simulink model "flightController"  (R2020b)
settings: Solver=ode3  StartTime=0.0  StopTime=10.0  FixedStep=Ts  RelTol=1e-3
undefined symbols (not defined in the file): DiscIntNeverNeededParam, Discrete, Estimator, g, init, Time, Ts
libraries: sharedtransform x3, pid_lib x2, aerolibconvert2 x1, ctrlSharedLib x1
settings Model: Creator=dbell44  LastModifiedBy=dbell44
settings OptimizationCC: DefaultParameterBehavior=Inlined  GainParamInheritBuiltInType=on  UseFloatMulNetSlope=on  DefaultUnderspecifiedDataType=single  UseSpecifiedMinMax=on  InlineInvariantSignals=on  PassReuseOutputArgsAs=Individual arguments  NoFixptDivByZeroProtection=on  EfficientFloat2IntCast=on  LifeSpan=1  OptimizeBlockOrder=speed  DifferentSizesBufferReuse=on  EfficientTunableParamExpr=on
settings DebuggingCC: ParameterTunabilityLossMsg=error  SFUnexpectedBacktrackingDiag=warning  SFNoUnconditionalDefaultTransitionDiag=warning
settings HardwareCC: ProdBitPerPointer=32  ProdBitPerSizeT=32  ProdBitPerPtrDiffT=32  ProdLargestAtomicInteger=Long  ProdLargestAtomicFloat=Double  ProdWordSize=32  ProdLongLongMode=on  ProdHWDeviceType=ARM Compatible->ARM Cortex-M
settings SFSimCC: MATLABDynamicMemAlloc=off
settings RTWCC: Description=Embedded Coder  SystemTargetFile=ert.tlc  GenCodeOnly=on  TemplateMakefile=ert_default_tmf  GenerateReport=on  BuildConfiguration=Faster Runs  LaunchReport=on  GenerateCodeMetricsReport=on
settings CodeAppCC: ForceParamTrailComments=on  IgnoreCustomStorageClasses=off  OperatorAnnotations=on  SimulinkDataObjDesc=on  SFDataObjDesc=on  CustomSymbolStrGlobalVar=rt$N$M  CustomSymbolStrType=$N$M  CustomSymbolStrFcn=$N$M$F  CustomSymbolStrMacro=$N$M  InsertBlockDesc=on  EnableCustomComments=on
settings ERTTargetCC: TargetLangStandard=C99 (ISO)  GenerateSampleERTMain=on  IncludeMdlTerminateFcn=off  CombineSignalStateStructs=on  SuppressErrorStatus=on  SupportAbsoluteTime=off  CodeInterfacePackaging=Reusable function  SupportNonFinite=off  SupportComplex=off  InlinedParameterPlacement=NonHierarchical  ERTCustomFileTemplate=example_file_process.tlc  ERTFilePackagingFormat=CompactWithDataFile

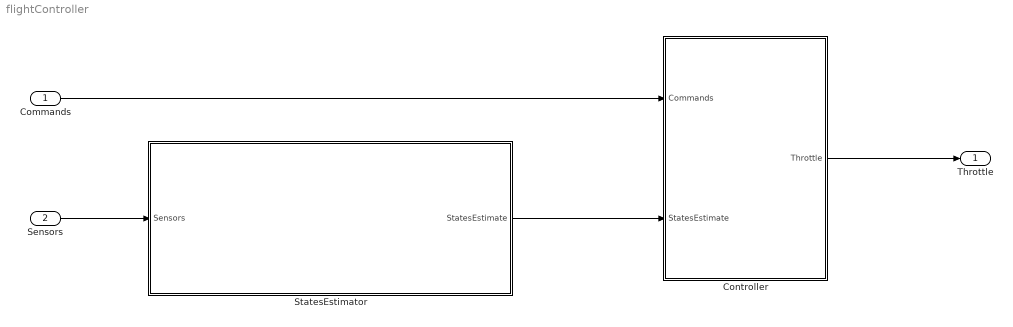
== system flightController ==
  Commands : Inport  OutDataTypeStr=Bus: command_t
  Sensors : Inport  Port=2  OutDataTypeStr=Bus: sensor_data_t
  Controller : Subsystem  TreatAsAtomicUnit=on
  StatesEstimator : Subsystem  TreatAsAtomicUnit=on
  Throttle : Outport
  wires:
  Sensors/1 -> StatesEstimator/1(Sensors)
  StatesEstimator/1(StatesEstimate) -> Controller/2(StatesEstimate)
  Commands/1 -> Controller/1(Commands)
  Controller/1(Throttle) -> Throttle/1

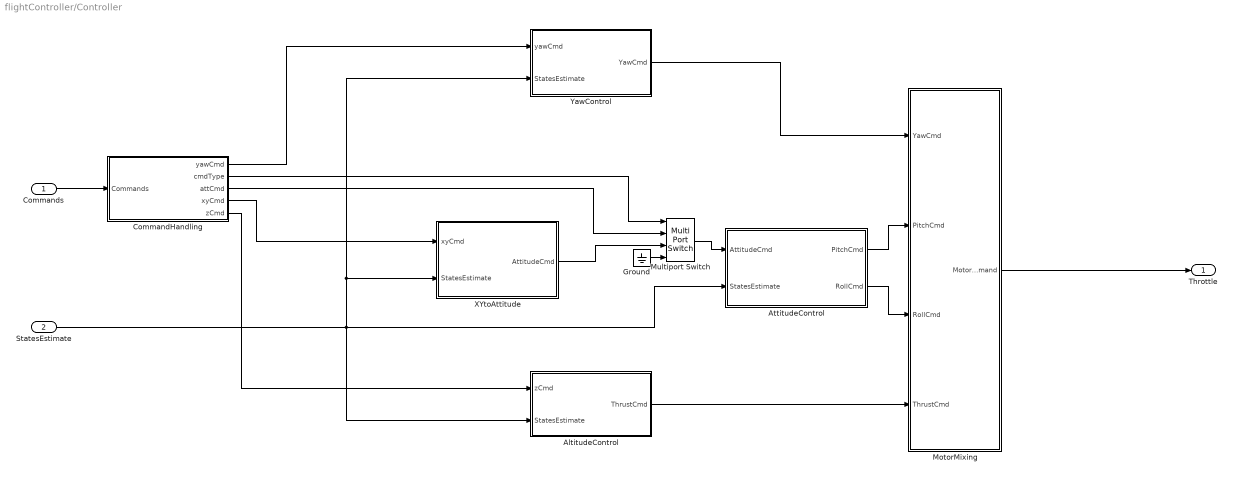
== system flightController/Controller ==
  Commands : Inport
  StatesEstimate : Inport  Port=2  OutDataTypeStr=Bus: states_estimate_t
  AltitudeControl : Subsystem
  AttitudeControl : Subsystem
  CommandHandling : Subsystem
  Ground : Ground
  MotorMixing : Subsystem
  Multiport Switch : MultiPortSwitch
  XYtoAttitude : Subsystem
  YawControl : Subsystem
  Throttle : Outport
  wires:
  StatesEstimate/1 -> YawControl/2(StatesEstimate), XYtoAttitude/2(StatesEstimate), AltitudeControl/2(StatesEstimate), AttitudeControl/2(StatesEstimate)
  AltitudeControl/1(ThrustCmd) -> MotorMixing/4(ThrustCmd)
  MotorMixing/1(MotorCommand) -> Throttle/1
  YawControl/1(YawCmd) -> MotorMixing/1(YawCmd)
  AttitudeControl/1(PitchCmd) -> MotorMixing/2(PitchCmd)
  AttitudeControl/2(RollCmd) -> MotorMixing/3(RollCmd)
  XYtoAttitude/1(AttitudeCmd) -> Multiport Switch/3
  Commands/1 -> CommandHandling/1(Commands)
  CommandHandling/1(yawCmd) -> YawControl/1(yawCmd)
  CommandHandling/5(zCmd) -> AltitudeControl/1(zCmd)
  CommandHandling/4(xyCmd) -> XYtoAttitude/1(xyCmd)
  CommandHandling/3(attCmd) -> Multiport Switch/2
  CommandHandling/2(cmdType) -> Multiport Switch/1
  Multiport Switch/1 -> AttitudeControl/1(AttitudeCmd)
  Ground/1 -> Multiport Switch/4

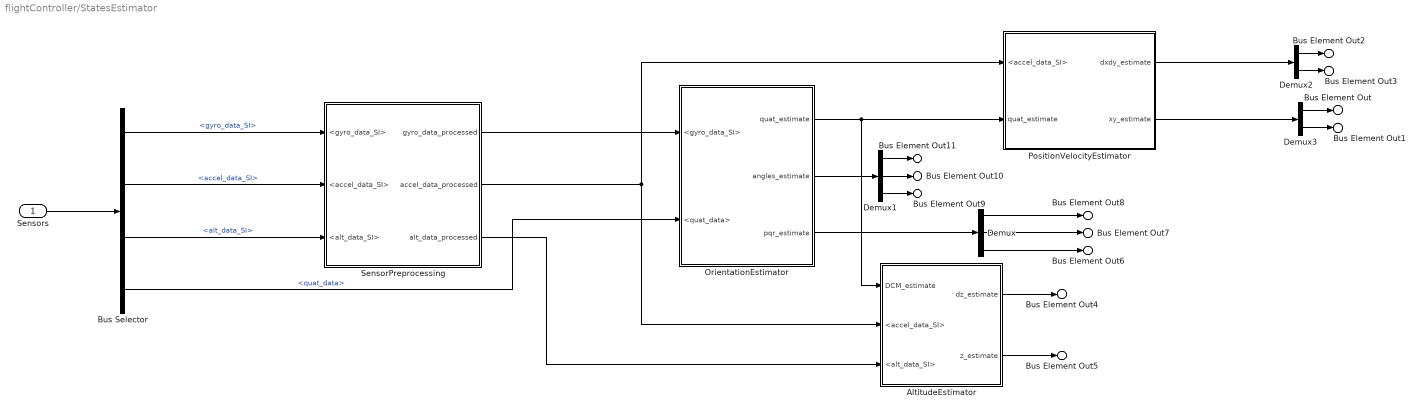
== system flightController/StatesEstimator ==
  Sensors : Inport  OutDataTypeStr=Bus: sensor_data_t
  AltitudeEstimator : Subsystem
  Bus Selector : BusSelector  OutputSignals=gyro_data_SI,accel_data_SI,alt_data_SI,quat_data
  Demux : Demux  Outputs=3
  Demux1 : Demux  Outputs=3
  Demux2 : Demux  Outputs=2
  Demux3 : Demux  Outputs=2
  OrientationEstimator : Subsystem
  PositionVelocityEstimator : Subsystem
  SensorPreprocessing : Subsystem
  Bus Element Out : Outport  PortName=StatesEstimate  Element=x
  Bus Element Out1 : Outport  PortName=StatesEstimate  Element=y
  Bus Element Out2 : Outport  PortName=StatesEstimate  Element=dx
  Bus Element Out3 : Outport  PortName=StatesEstimate  Element=dy
  Bus Element Out4 : Outport  PortName=StatesEstimate  Element=dz
  Bus Element Out5 : Outport  PortName=StatesEstimate  Element=z
  Bus Element Out6 : Outport  PortName=StatesEstimate  Element=r
  Bus Element Out7 : Outport  PortName=StatesEstimate  Element=q
  Bus Element Out8 : Outport  PortName=StatesEstimate  Element=p
  Bus Element Out9 : Outport  PortName=StatesEstimate  Element=roll
  Bus Element Out10 : Outport  PortName=StatesEstimate  Element=pitch
  Bus Element Out11 : Outport  PortName=StatesEstimate  Element=yaw
  wires:
  Sensors/1 -> Bus Selector/1
  Bus Selector/3 -> SensorPreprocessing/3(<alt_data_SI>)  "<alt_data_SI>"
  PositionVelocityEstimator/1(dxdy_estimate) -> Demux2/1
  PositionVelocityEstimator/2(xy_estimate) -> Demux3/1
  OrientationEstimator/1(quat_estimate) -> AltitudeEstimator/1(DCM_estimate), PositionVelocityEstimator/2(quat_estimate)
  Bus Selector/1 -> SensorPreprocessing/1(<gyro_data_SI>)  "<gyro_data_SI>"
  OrientationEstimator/2(angles_estimate) -> Demux1/1
  Demux1/2 -> Bus Element Out10/1
  AltitudeEstimator/2(z_estimate) -> Bus Element Out5/1
  Demux3/1 -> Bus Element Out/1
  Demux3/2 -> Bus Element Out1/1
  Demux2/1 -> Bus Element Out2/1
  Demux2/2 -> Bus Element Out3/1
  Demux1/3 -> Bus Element Out9/1
  Demux1/1 -> Bus Element Out11/1
  OrientationEstimator/3(pqr_estimate) -> Demux/1
  Demux/1 -> Bus Element Out8/1
  Demux/2 -> Bus Element Out7/1
  Demux/3 -> Bus Element Out6/1
  SensorPreprocessing/2(accel_data_processed) -> AltitudeEstimator/2(<accel_data_SI>), PositionVelocityEstimator/1(<accel_data_SI>)
  Bus Selector/2 -> SensorPreprocessing/2(<accel_data_SI>)  "<accel_data_SI>"
  SensorPreprocessing/1(gyro_data_processed) -> OrientationEstimator/1(<gyro_data_SI>)
  SensorPreprocessing/3(alt_data_processed) -> AltitudeEstimator/3(<alt_data_SI>)
  Bus Selector/4 -> OrientationEstimator/2(<quat_data>)  "<quat_data>"
  AltitudeEstimator/1(dz_estimate) -> Bus Element Out4/1

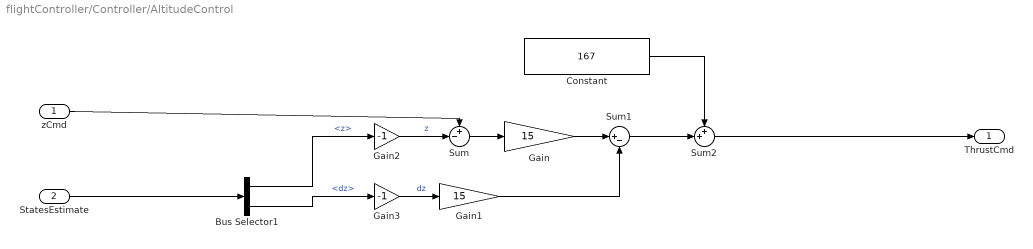
== system flightController/Controller/AltitudeControl ==
  zCmd : Inport
  StatesEstimate : Inport  Port=2
  Bus Selector1 : BusSelector  OutputSignals=z,dz
  Constant : Constant  Value=167
  Gain : Gain  Gain=15
  Gain1 : Gain  Gain=15
  Gain2 : Gain  Gain=-1
  Gain3 : Gain  Gain=-1
  Sum : Sum  Inputs=+-|
  Sum1 : Sum  Inputs=|+-
  Sum2 : Sum  Inputs=++|
  ThrustCmd : Outport
  wires:
  Gain3/1 -> Gain1/1  "dz"
  Bus Selector1/1 -> Gain2/1  "<z>"
  Gain2/1 -> Sum/2  "z"
  Gain1/1 -> Sum1/2
  Constant/1 -> Sum2/1
  Sum2/1 -> ThrustCmd/1
  Sum/1 -> Gain/1
  Bus Selector1/2 -> Gain3/1  "<dz>"
  Gain/1 -> Sum1/1
  StatesEstimate/1 -> Bus Selector1/1
  zCmd/1 -> Sum/1
  Sum1/1 -> Sum2/2

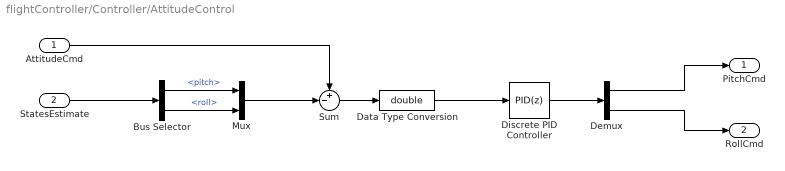
== system flightController/Controller/AttitudeControl ==
  AttitudeCmd : Inport
  StatesEstimate : Inport  Port=2
  Bus Selector : BusSelector  OutputSignals=pitch,roll
  Data Type Conversion : DataTypeConversion  OutDataTypeStr=double
  Demux : Demux  Outputs=2
  Discrete PID Controller : pid_lib/PID Controller  Controller=PID  Form=Parallel  TimeDomain=Discrete-time  UseExternalTs=off  SampleTime=-1  IntegratorMethod=Forward Euler  FilterMethod=Forward Euler  ControllerParametersSource=internal  P=5  I=5  D=3  UseFilter=off  N=100  TunerSelectOption=Transfer Function Based (PID Tuner App)  InitialConditionSource=internal  InitialConditionForIntegrator=0  InitialConditionForFilter=0  DifferentiatorICPrevScaledInput=0  ExternalReset=none  TrackingMode=off  Kt=1  LimitOutput=off  SatLimitsSource=internal  UpperSaturationLimit=inf  LowerSaturationLimit=-inf  LinearizeAsGain=off  AntiWindupMode=none  Kb=1  POutMin=[]  POutMax=[]  IOutMin=[]  IOutMax=[]  DOutMin=[]  DOutMax=[]  NOutMin=[]  NOutMax=[]  SumOutMin=[]  SumOutMax=[]  SaturationOutMin=[]  SaturationOutMax=[]  PParamMin=[]  PParamMax=[]  IParamMin=[]  IParamMax=[]  DParamMin=[]  DParamMax=[]  NParamMin=[]  NParamMax=[]  KbParamMin=[]  KbParamMax=[]  KtParamMin=[]  KtParamMax=[]  KbOutMin=[]  KbOutMax=[]  KtOutMin=[]  KtOutMax=[]  IntegratorOutMin=[]  IntegratorOutMax=[]  FilterOutMin=[]  FilterOutMax=[]  SumI1OutMin=[]  SumI1OutMax=[]  SumI2OutMin=[]  SumI2OutMax=[]  SumI3OutMin=[]  SumI3OutMax=[]  SumI4OutMin=[]  SumI4OutMax=[]  SumDOutMin=[]  SumDOutMax=[]  DifferentiatorOutMin=[]  DifferentiatorOutMax=[]  FilterDiffOutCoefMin=[]  FilterDiffOutCoefMax=[]  ReciprocalOutMin=[]  ReciprocalOutMax=[]  SumDenOutMin=[]  SumDenOutMax=[]  SumNumOutMin=[]  SumNumOutMax=[]  DivideOutMin=[]  DivideOutMax=[]  UdiffTsProdOutMin=[]  UdiffTsProdOutMax=[]  NTsProdOutMin=[]  NTsProdOutMax=[]  UintegralTsProdOutMin=[]  UintegralTsProdOutMax=[]  UngainTsProdOutMin=[]  UngainTsProdOutMax=[]  IntegratorContinuousStateAttributes=''  IntegratorStateMustResolveToSignalObject=off  IntegratorRTWStateStorageClass=Auto  FilterContinuousStateAttributes=''  FilterStateMustResolveToSignalObject=off  FilterRTWStateStorageClass=Auto  ParallelPVariant=InternalParameters  IdealPVariant=Disabled  IVariant=InternalParameters  DVariant=InternalParameters  IntegratorVariant=Discrete  SatVariant=Disabled  AWVariant=Passthrough  PCopyVariant=Disabled  TRVariant=Disabled  FdbkBlocksVariant=Forward  IdealPFdbkVariant=Disabled  SatFdbkVariant=Disabled  DerivativeFilterVariant=Differentiator  NVariant=Passthrough  NCopyVariant=Disabled_SignalSpec  FilterICVariant=InternalICsDifferentiator  IntegratorICVariant=InternalICs  ExternalResetVariant=Disabled  TRSumVariant=Passthrough  SumFdbkVariant=Disabled  SumVariant=Sum_PID  TsampFilterVariant=InternalTs  TsampNgainVariant=Passthrough  TsampIntegralVariant=Passthrough  ExternalSaturationOutDataTypeStr=Inherit: Same as second input
  Mux : Mux  Inputs=2
  Sum : Sum  Inputs=+-|
  PitchCmd : Outport
  RollCmd : Outport  Port=2
  wires:
  AttitudeCmd/1 -> Sum/1
  StatesEstimate/1 -> Bus Selector/1
  Bus Selector/2 -> Mux/2  "<roll>"
  Bus Selector/1 -> Mux/1  "<pitch>"
  Sum/1 -> Data Type Conversion/1
  Discrete PID Controller/1 -> Demux/1
  Data Type Conversion/1 -> Discrete PID Controller/1
  Mux/1 -> Sum/2
  Demux/1 -> PitchCmd/1
  Demux/2 -> RollCmd/1

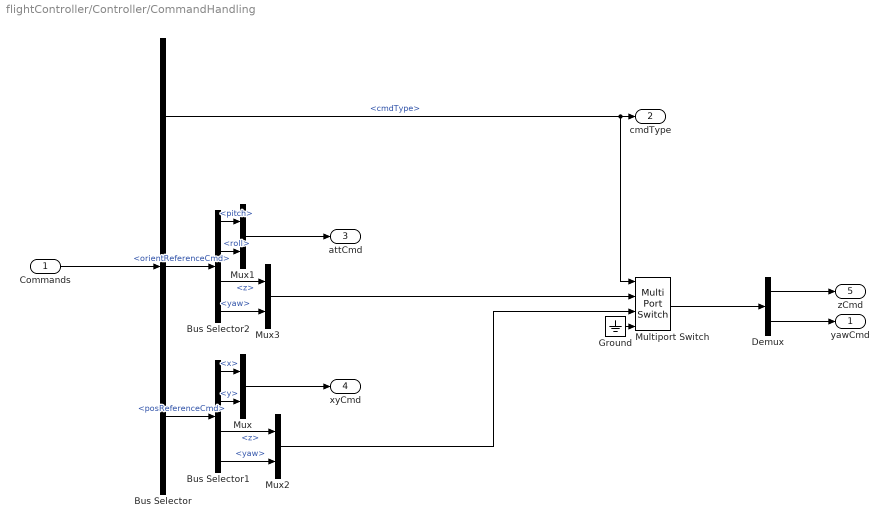
== system flightController/Controller/CommandHandling ==
  Commands : Inport
  Bus Selector : BusSelector  OutputSignals=cmdType,orientReferenceCmd,posReferenceCmd
  Bus Selector1 : BusSelector  OutputSignals=x,y,z,yaw
  Bus Selector2 : BusSelector  OutputSignals=pitch,roll,z,yaw
  Demux : Demux  Outputs=2
  Ground : Ground
  Multiport Switch : MultiPortSwitch
  Mux{,1..3} (4 alike) : Mux  Inputs=2
  yawCmd : Outport
  cmdType : Outport  Port=2
  attCmd : Outport  Port=3
  xyCmd : Outport  Port=4
  zCmd : Outport  Port=5
  wires:
  Commands/1 -> Bus Selector/1
  Bus Selector/1 -> Multiport Switch/1, cmdType/1  "<cmdType>"
  Bus Selector1/1 -> Mux/1  "<x>"
  Bus Selector1/2 -> Mux/2  "<y>"
  Mux/1 -> xyCmd/1
  Bus Selector1/3 -> Mux2/1  "<z>"
  Bus Selector1/4 -> Mux2/2  "<yaw>"
  Bus Selector2/1 -> Mux1/1  "<pitch>"
  Bus Selector2/2 -> Mux1/2  "<roll>"
  Mux1/1 -> attCmd/1
  Multiport Switch/1 -> Demux/1
  Demux/2 -> yawCmd/1
  Demux/1 -> zCmd/1
  Bus Selector2/3 -> Mux3/1  "<z>"
  Bus Selector2/4 -> Mux3/2  "<yaw>"
  Mux3/1 -> Multiport Switch/2
  Mux2/1 -> Multiport Switch/3
  Bus Selector/3 -> Bus Selector1/1  "<posReferenceCmd>"
  Bus Selector/2 -> Bus Selector2/1  "<orientReferenceCmd>"
  Ground/1 -> Multiport Switch/4

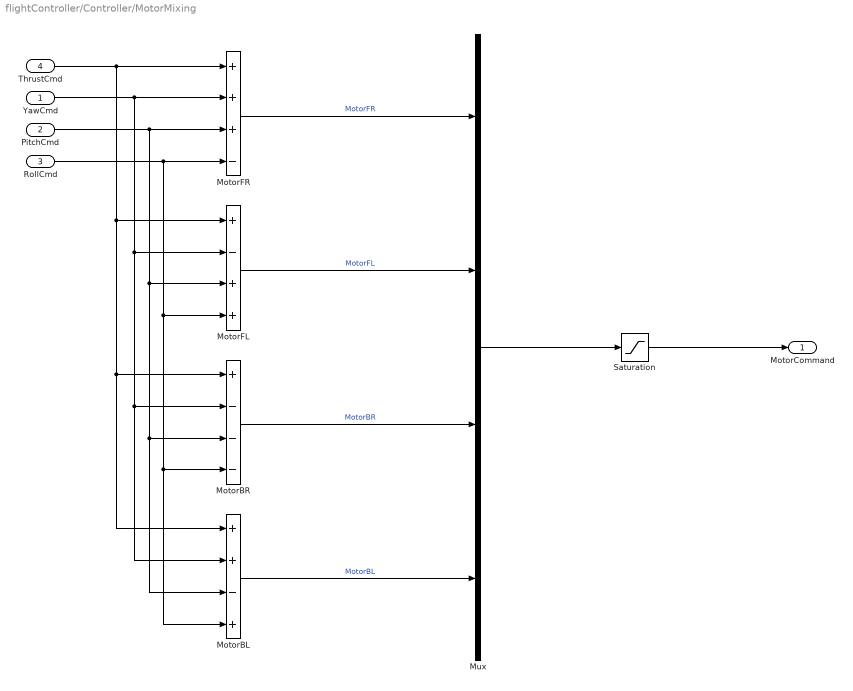
== system flightController/Controller/MotorMixing ==
  YawCmd : Inport
  PitchCmd : Inport  Port=2
  RollCmd : Inport  Port=3
  ThrustCmd : Inport  Port=4
  MotorBL : Sum  Inputs=++-+
  MotorBR : Sum  Inputs=+---
  MotorFL : Sum  Inputs=+-++
  MotorFR : Sum  Inputs=+++-
  Mux : Mux
  Saturation : Saturate  UpperLimit=1000  LowerLimit=0
  MotorCommand : Outport
  wires:
  ThrustCmd/1 -> MotorBL/1, MotorBR/1, MotorFL/1, MotorFR/1
  YawCmd/1 -> MotorBL/2, MotorBR/2, MotorFL/2, MotorFR/2
  PitchCmd/1 -> MotorBL/3, MotorBR/3, MotorFL/3, MotorFR/3
  RollCmd/1 -> MotorBL/4, MotorBR/4, MotorFL/4, MotorFR/4
  MotorFR/1 -> Mux/1  "MotorFR"
  MotorFL/1 -> Mux/2  "MotorFL"
  MotorBR/1 -> Mux/3  "MotorBR"
  MotorBL/1 -> Mux/4  "MotorBL"
  Mux/1 -> Saturation/1
  Saturation/1 -> MotorCommand/1

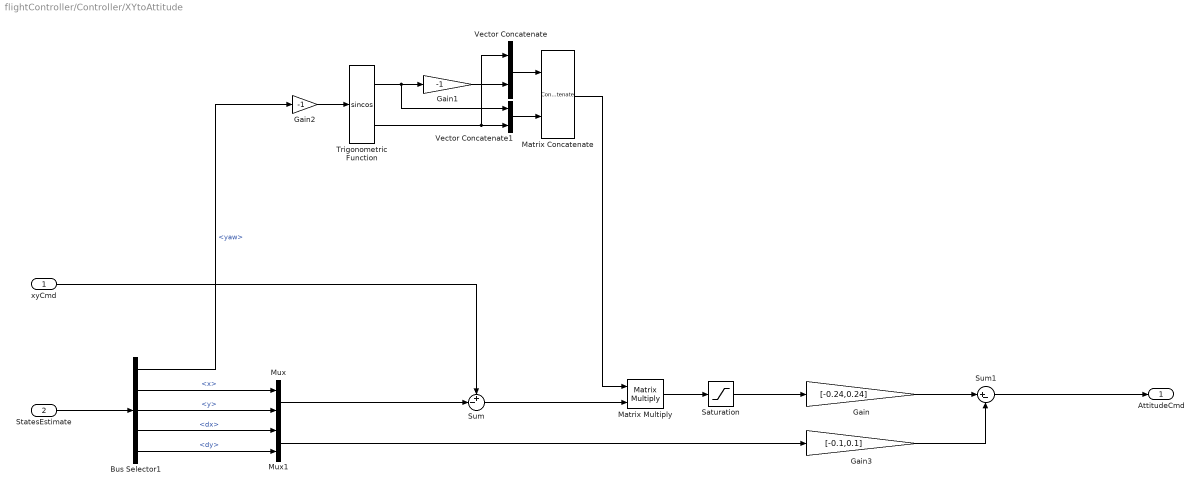
== system flightController/Controller/XYtoAttitude ==
  xyCmd : Inport
  StatesEstimate : Inport  Port=2
  Bus Selector1 : BusSelector  OutputSignals=yaw,x,y,dx,dy
  Gain : Gain  Gain=[-0.24,0.24]
  Gain1 : Gain  Gain=-1
  Gain2 : Gain  Gain=-1
  Gain3 : Gain  Gain=[-0.1,0.1]
  Matrix Concatenate : Concatenate  Mode=Multidimensional array  ConcatenateDimension=2
  Matrix Multiply : Product  Multiplication=Matrix(*)
  Mux : Mux  Inputs=2
  Mux1 : Mux  Inputs=2
  Saturation : Saturate  UpperLimit=3  LowerLimit=-3  OutDataTypeStr=single
  Sum : Sum  Inputs=+-|
  Sum1 : Sum  Inputs=|+-
  Trigonometric Function : Trigonometry  Operator=sincos
  Vector Concatenate : Concatenate
  Vector Concatenate1 : Concatenate
  AttitudeCmd : Outport  VectorParamsAs1DForOutWhenUnconnected=off
  wires:
  StatesEstimate/1 -> Bus Selector1/1
  Bus Selector1/2 -> Mux/1  "<x>"
  Bus Selector1/3 -> Mux/2  "<y>"
  Bus Selector1/1 -> Gain2/1  "<yaw>"
  Vector Concatenate/1 -> Matrix Concatenate/1
  Vector Concatenate1/1 -> Matrix Concatenate/2
  Trigonometric Function/1 -> Gain1/1, Vector Concatenate1/1
  Trigonometric Function/2 -> Vector Concatenate1/2, Vector Concatenate/1
  Gain1/1 -> Vector Concatenate/2
  Gain2/1 -> Trigonometric Function/1
  Mux/1 -> Sum/2
  Sum/1 -> Matrix Multiply/2
  Matrix Concatenate/1 -> Matrix Multiply/1
  xyCmd/1 -> Sum/1
  Sum1/1 -> AttitudeCmd/1
  Bus Selector1/4 -> Mux1/1  "<dx>"
  Bus Selector1/5 -> Mux1/2  "<dy>"
  Matrix Multiply/1 -> Saturation/1
  Mux1/1 -> Gain3/1
  Gain/1 -> Sum1/1
  Gain3/1 -> Sum1/2
  Saturation/1 -> Gain/1

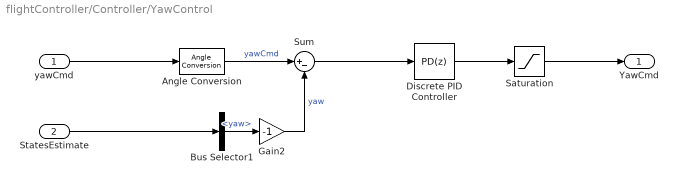
== system flightController/Controller/YawControl ==
  yawCmd : Inport
  StatesEstimate : Inport  Port=2
  Angle Conversion : aerolibconvert2/Angle Conversion  IU=deg  OU=rad
  Bus Selector1 : BusSelector  OutputSignals=yaw
  Discrete PID Controller : pid_lib/PID Controller  Controller=PD  Form=Parallel  TimeDomain=Discrete-time  UseExternalTs=off  SampleTime=-1  IntegratorMethod=Forward Euler  FilterMethod=Forward Euler  ControllerParametersSource=internal  P=200  I=50  D=30  UseFilter=off  N=100  TunerSelectOption=Transfer Function Based (PID Tuner App)  InitialConditionSource=internal  InitialConditionForIntegrator=0  InitialConditionForFilter=0  DifferentiatorICPrevScaledInput=0  ExternalReset=none  TrackingMode=off  Kt=1  LimitOutput=off  SatLimitsSource=internal  UpperSaturationLimit=inf  LowerSaturationLimit=-inf  LinearizeAsGain=off  AntiWindupMode=none  Kb=1  PGainOutDataTypeStr=single  PProdOutDataTypeStr=single  POutMin=[]  POutMax=[]  IOutMin=[]  IOutMax=[]  DGainOutDataTypeStr=single  DProdOutDataTypeStr=single  DOutMin=[]  DOutMax=[]  NGainOutDataTypeStr=single  NProdOutDataTypeStr=single  NOutMin=[]  NOutMax=[]  SumOutDataTypeStr=single  SumOutMin=[]  SumOutMax=[]  SaturationOutMin=[]  SaturationOutMax=[]  PParamDataTypeStr=single  PParamMin=[]  PParamMax=[]  IParamMin=[]  IParamMax=[]  DParamDataTypeStr=single  DParamMin=[]  DParamMax=[]  NParamDataTypeStr=single  NParamMin=[]  NParamMax=[]  KbParamMin=[]  KbParamMax=[]  KtParamMin=[]  KtParamMax=[]  KbOutMin=[]  KbOutMax=[]  KtOutMin=[]  KtOutMax=[]  IntegratorOutMin=[]  IntegratorOutMax=[]  FilterOutDataTypeStr=single  FilterOutMin=[]  FilterOutMax=[]  SumI1OutMin=[]  SumI1OutMax=[]  SumI2OutMin=[]  SumI2OutMax=[]  SumI3OutMin=[]  SumI3OutMax=[]  SumI4OutMin=[]  SumI4OutMax=[]  SumDOutDataTypeStr=single  SumDOutMin=[]  SumDOutMax=[]  SumAccumDataTypeStr=single  SumDAccumDataTypeStr=single  DifferentiatorOutMin=[]  DifferentiatorOutMax=[]  FilterDiffOutCoefMin=[]  FilterDiffOutCoefMax=[]  ReciprocalOutMin=[]  ReciprocalOutMax=[]  SumDenOutMin=[]  SumDenOutMax=[]  SumNumOutMin=[]  SumNumOutMax=[]  DivideOutMin=[]  DivideOutMax=[]  UdiffTsProdOutMin=[]  UdiffTsProdOutMax=[]  NTsProdOutMin=[]  NTsProdOutMax=[]  UintegralTsProdOutMin=[]  UintegralTsProdOutMax=[]  UngainTsProdOutMin=[]  UngainTsProdOutMax=[]  IntegratorContinuousStateAttributes=''  IntegratorStateMustResolveToSignalObject=off  IntegratorRTWStateStorageClass=Auto  FilterContinuousStateAttributes=''  FilterStateMustResolveToSignalObject=off  FilterRTWStateStorageClass=Auto  ParallelPVariant=InternalParameters  IdealPVariant=Disabled  IVariant=Disabled  DVariant=InternalParameters  IntegratorVariant=Disabled  SatVariant=Disabled  AWVariant=Disabled  PCopyVariant=Disabled  TRVariant=Disabled  FdbkBlocksVariant=Forward  IdealPFdbkVariant=Disabled  SatFdbkVariant=Disabled  DerivativeFilterVariant=Differentiator  NVariant=Passthrough  NCopyVariant=Disabled_SignalSpec  FilterICVariant=InternalICsDifferentiator  IntegratorICVariant=Disabled  ExternalResetVariant=Disabled  TRSumVariant=Passthrough  SumFdbkVariant=Disabled  SumVariant=Sum_PD  TsampFilterVariant=InternalTs  TsampNgainVariant=Passthrough  TsampIntegralVariant=Disabled_SignalSpec  ExternalSaturationOutDataTypeStr=Inherit: Same as second input
  Gain2 : Gain  Gain=-1
  Saturation : Saturate  UpperLimit=150  LowerLimit=-150
  Sum : Sum  Inputs=|+-
  YawCmd : Outport
  wires:
  Gain2/1 -> Sum/2  "yaw"
  Sum/1 -> Discrete PID Controller/1
  Bus Selector1/1 -> Gain2/1  "<yaw>"
  Angle Conversion/1 -> Sum/1  "yawCmd"
  StatesEstimate/1 -> Bus Selector1/1
  Discrete PID Controller/1 -> Saturation/1
  Saturation/1 -> YawCmd/1
  yawCmd/1 -> Angle Conversion/1

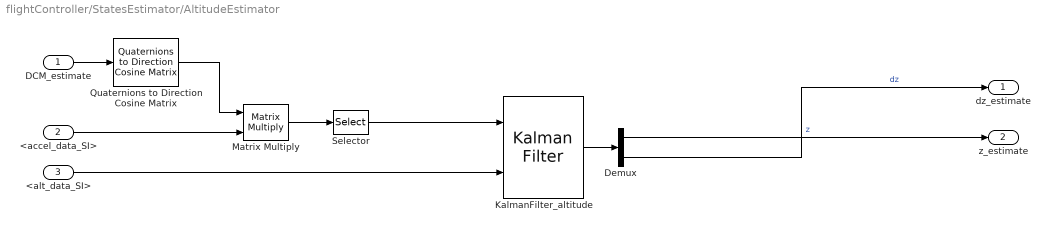
== system flightController/StatesEstimator/AltitudeEstimator ==
  DCM_estimate : Inport
  <accel_data_SI> : Inport  Port=2
  <alt_data_SI> : Inport  Port=3
  Demux : Demux  Outputs=2
  KalmanFilter_altitude : ctrlSharedLib/Kalman Filter  TimeDomain=Discrete-Time  UseCurrentEstimator=on  ModelSource=Individual A, B, C, D matrices  ModelSourceVariable=sys  A=[1 Ts; 0 1]  B=[0;Ts]  C=[1 0]  D=[0]  NumberOfStates=2  NumberOfInputs=2  NumberOfOutputs=2  InitialEstimateSource=Dialog  X0=[init.posNED(3) 0]  P0=10  UseK=off  UseGH=on  NumberOfProcessNoiseInputs=2  G=Estimator.alt.kf.G  TimeInvariantG=on  H=Estimator.alt.kf.H  TimeInvariantH=on  Q=Estimator.alt.kf.Q  TimeInvariantQ=on  R=Estimator.alt.kf.R  TimeInvariantR=on  N=Estimator.alt.kf.N  TimeInvariantN=on  AddInputPort=on  AddEnablePort=off  OutputEstimatedY=off  OutputP=off  Ts=-1
  Matrix Multiply : Product  Multiplication=Matrix(*)  OutDataTypeStr=single
  Quaternions to Direction Cosine Matrix : sharedtransform/Quaternions to  Direction Cosine Matrix  aMode=aMode
      settings: SourceProductBaseCode=AE,PW,MT,UV,VE,VP
  Selector : Selector  InputPortWidth=3  IndexOptions=Index vector (dialog)  Indices=[3]  OutputSizes=1
  dz_estimate : Outport
  z_estimate : Outport  Port=2
  wires:
  <alt_data_SI>/1 -> KalmanFilter_altitude/2
  KalmanFilter_altitude/1 -> Demux/1
  Demux/1 -> z_estimate/1  "z"
  <accel_data_SI>/1 -> Matrix Multiply/2
  Demux/2 -> dz_estimate/1  "dz"
  DCM_estimate/1 -> Quaternions to Direction Cosine Matrix/1
  Matrix Multiply/1 -> Selector/1
  Selector/1 -> KalmanFilter_altitude/1
  Quaternions to Direction Cosine Matrix/1 -> Matrix Multiply/1

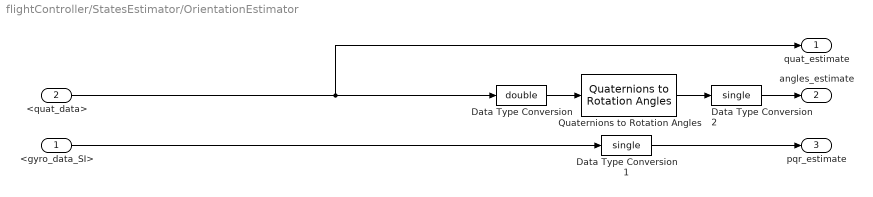
== system flightController/StatesEstimator/OrientationEstimator ==
  <gyro_data_SI> : Inport
  <quat_data> : Inport  Port=2
  Data Type Conversion : DataTypeConversion  OutDataTypeStr=double
  Data Type Conversion1 : DataTypeConversion  OutDataTypeStr=single
  Data Type Conversion2 : DataTypeConversion  OutDataTypeStr=single
  Quaternions to Rotation Angles : sharedtransform/Quaternions to Rotation Angles  rotationOrder=ZYX  aMode=aMode
      settings: SourceProductBaseCode=AE,PW,MT,UV,VE,VP
  quat_estimate : Outport
  angles_estimate : Outport  Port=2
  pqr_estimate : Outport  Port=3
  wires:
  <gyro_data_SI>/1 -> Data Type Conversion1/1
  Quaternions to Rotation Angles/1 -> Data Type Conversion2/1
  Data Type Conversion/1 -> Quaternions to Rotation Angles/1
  Data Type Conversion1/1 -> pqr_estimate/1
  Data Type Conversion2/1 -> angles_estimate/1
  <quat_data>/1 -> Data Type Conversion/1, quat_estimate/1

== system flightController/StatesEstimator/PositionVelocityEstimator ==
  <accel_data_SI> : Inport
  quat_estimate : Inport  Port=2
  PositionEstimator : Subsystem
  VelocityEstimator : Subsystem
  dxdy_estimate : Outport
  xy_estimate : Outport  Port=2
  wires:
  VelocityEstimator/1(dxdy_estimate) -> dxdy_estimate/1, PositionEstimator/1(dxdy_estimate)
  quat_estimate/1 -> VelocityEstimator/1(quat_estimate)
  <accel_data_SI>/1 -> VelocityEstimator/2(<accel_data_SI>)
  PositionEstimator/1(xy_estimate) -> xy_estimate/1

== system flightController/StatesEstimator/SensorPreprocessing ==
  <gyro_data_SI> : Inport
  <accel_data_SI> : Inport  Port=2
  <alt_data_SI> : Inport  Port=3
  gyro_data_processed : Outport
  accel_data_processed : Outport  Port=2
  alt_data_processed : Outport  Port=3
  wires:
  <gyro_data_SI>/1 -> gyro_data_processed/1
  <accel_data_SI>/1 -> accel_data_processed/1
  <alt_data_SI>/1 -> alt_data_processed/1

== system flightController/StatesEstimator/PositionVelocityEstimator/PositionEstimator ==
  dxdy_estimate : Inport
  Discrete-Time Integrator : DiscreteIntegrator  SampleTime=Ts  ICPrevOutput=DiscIntNeverNeededParam  ICPrevScaledInput=DiscIntNeverNeededParam
  xy_estimate : Outport
  wires:
  Discrete-Time Integrator/1 -> xy_estimate/1
  dxdy_estimate/1 -> Discrete-Time Integrator/1

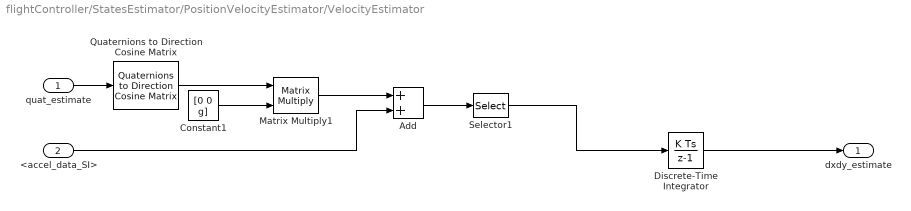
== system flightController/StatesEstimator/PositionVelocityEstimator/VelocityEstimator ==
  quat_estimate : Inport
  <accel_data_SI> : Inport  Port=2
  Add : Sum
  Constant1 : Constant  Value=[0 0 g]
  Discrete-Time Integrator : DiscreteIntegrator  SampleTime=Ts  ICPrevOutput=DiscIntNeverNeededParam  ICPrevScaledInput=DiscIntNeverNeededParam
  Matrix Multiply1 : Product  Multiplication=Matrix(*)  OutDataTypeStr=single
  Quaternions to Direction Cosine Matrix : sharedtransform/Quaternions to  Direction Cosine Matrix  aMode=aMode
      settings: SourceProductBaseCode=AE,PW,MT,UV,VE,VP
  Selector1 : Selector  InputPortWidth=3  IndexOptions=Index vector (dialog)  Indices=[1 2]  OutputSizes=1
  dxdy_estimate : Outport
  wires:
  Discrete-Time Integrator/1 -> dxdy_estimate/1
  Selector1/1 -> Discrete-Time Integrator/1
  Matrix Multiply1/1 -> Add/1
  Constant1/1 -> Matrix Multiply1/2
  quat_estimate/1 -> Quaternions to Direction Cosine Matrix/1
  Add/1 -> Selector1/1
  <accel_data_SI>/1 -> Add/2
  Quaternions to Direction Cosine Matrix/1 -> Matrix Multiply1/1
